simulink model "SWC_FDC_type"  (R2021b)
settings: Solver=FixedStepDiscrete  StartTime=0.0  StopTime=10.0  FixedStep=0.001  RelTol=1e-3
values from neighbouring files (symbols this model uses):
  DID_VCUKey = uint16(0x0202)    [vcu_local_hdr.m]
  DID_XWD = uint16(513)    [vcu_local_hdr.m]
  DIDLen_DKCKey = uint16(8)    [vcu_local_hdr.m]
  DIDLen_DynoMode = uint16(1)    [vcu_local_hdr.m]
  DIDLen_LFLowPresThre = uint16(1)    [vcu_local_hdr.m]
  DIDLen_LFSensorID = uint16(4)    [vcu_local_hdr.m]
  DIDLen_LRLowPresThre = uint16(1)    [vcu_local_hdr.m]
  DIDLen_LRSensorID = uint16(4)    [vcu_local_hdr.m]
  DIDLen_RFLowPresThre = uint16(1)    [vcu_local_hdr.m]
  DIDLen_RFSensorID = uint16(4)    [vcu_local_hdr.m]
  DIDLen_RRLowPresThre = uint16(1)    [vcu_local_hdr.m]
  DIDLen_RRSensorID = uint16(4)    [vcu_local_hdr.m]
  DIDLen_SensorMode = uint16(1)    [vcu_local_hdr.m]
  DIDLen_TPMSLearnSta = uint16(1)    [vcu_local_hdr.m]
  DIDLen_WhlPres = uint16(4)    [vcu_local_hdr.m]
  DIDLen_WhlSensorBattSta = uint16(1)    [vcu_local_hdr.m]
  DIDLen_WhlTmp = uint16(4)    [vcu_local_hdr.m]
  DIDLen_XWDMode = uint16(1)    [vcu_local_hdr.m]
  DIDNum_DKCKey = uint16(0x0202)    [vcu_local_hdr.m]
  DIDNum_DynoMode = uint16(0x0203)    [vcu_local_hdr.m]
  DIDNum_LFLowPresThre = uint16(0x0B08)    [vcu_local_hdr.m]
  DIDNum_LFSensorID = uint16(0x0B01)    [vcu_local_hdr.m]
  DIDNum_LRLowPresThre = uint16(0x0B0A)    [vcu_local_hdr.m]
  DIDNum_LRSensorID = uint16(0x0B03)    [vcu_local_hdr.m]
  DIDNum_RFLowPresThre = uint16(0x0B09)    [vcu_local_hdr.m]
  DIDNum_RFSensorID = uint16(0x0B02)    [vcu_local_hdr.m]
  DIDNum_RRLowPresThre = uint16(0x0B0B)    [vcu_local_hdr.m]
  DIDNum_RRSensorID = uint16(0x0B04)    [vcu_local_hdr.m]
  DIDNum_SensorMode = uint16(0x0B0C)    [vcu_local_hdr.m]
  DIDNum_TPMSLearnSta = uint16(0x0B0D)    [vcu_local_hdr.m]
  DIDNum_WhlPres = uint16(0x0B05)    [vcu_local_hdr.m]
  DIDNum_WhlSensorBattSta = uint16(0x0B07)    [vcu_local_hdr.m]
  DIDNum_WhlTmp = uint16(0x0B06)    [vcu_local_hdr.m]
  DIDNum_XWDMode = uint16(0x0201)    [vcu_local_hdr.m]
  DIDVCUKeyLength = uint16(8)    [vcu_local_hdr.m]
  ENUM_DRIVETRAIN_AWD = uint8(  2  )    [vcu_local_hdr.m]
  ENUM_DRIVETRAIN_FWD = uint8(  1  )    [vcu_local_hdr.m]
  ENUM_DRIVETRAIN_RWD = uint8(  0  )    [vcu_local_hdr.m]
  ENUM_TPMSLearnStatus_LEARNED = uint8(  1  )    [vcu_local_hdr.m]
  ENUM_TPMSLearnStatus_LEARNFAIL = uint8(  2  )    [vcu_local_hdr.m]
  ENUM_TPMSLearnStatus_NOTLEARN = uint8(  0  )    [vcu_local_hdr.m]
  ENUM_TPMSSTA_FAT = uint8(  8  )    [vcu_local_hdr.m]
  ENUM_TPMSSTA_LOWBATTERY = uint8(  2  )    [vcu_local_hdr.m]
  FALSE = boolean( 0 )    [vcu_local_hdr.m]
  ONE_INT = uint8(1)    [vcu_local_hdr.m]
  P_boolean = 0.0    [APPTypes.sldd]
  TRUE = boolean( 1 )    [vcu_local_hdr.m]
  ZERO_FLOAT = single(0)    [vcu_local_hdr.m]
  ZERO_INT = uint8(0)    [vcu_local_hdr.m]
undefined symbols (not defined in the file or in its folder): f32_ApsOutVehSpdSig, KHAL_DKCDecryptEnable_flg_ovrdflg, KHAL_DKCDecryptEnable_flg_ovrdval, KHAL_RandomNumberY1_enum, KHAL_RandomNumberY2_enum, KHAL_RandomNumberY_ovrdflg, KHAL_TPMSRESBUTT_flg_ovrdflg, KHAL_TPMSRESBUTT_flg_ovrdval, R_DIDWriteCDD_CSOP_DIDSet_DKCKey, R_DIDWriteCDD_CSOP_DIDSet_DynoMode, R_DIDWriteCDD_CSOP_DIDSet_LFLowPresThre, R_DIDWriteCDD_CSOP_DIDSet_LFSensorID, R_DIDWriteCDD_CSOP_DIDSet_LRLowPresThre, R_DIDWriteCDD_CSOP_DIDSet_LRSensorID, R_DIDWriteCDD_CSOP_DIDSet_RFLowPresThre, R_DIDWriteCDD_CSOP_DIDSet_RFSensorID, R_DIDWriteCDD_CSOP_DIDSet_RRLowPresThre, R_DIDWriteCDD_CSOP_DIDSet_RRSensorID, R_DIDWriteCDD_CSOP_DIDSet_SensorMode, R_DIDWriteCDD_CSOP_DIDSet_TPMSLearnSta, R_DIDWriteCDD_CSOP_DIDSet_WhlPres, R_DIDWriteCDD_CSOP_DIDSet_WhlSensorBattSta, R_DIDWriteCDD_CSOP_DIDSet_WhlTmp, R_DIDWriteCDD_CSOP_DIDSet_XWDMode, R_E2E_CAN3_VCU1_CSOP_Write_CAN3_VCU1, R_E2E_CAN4_VCU1_CSOP_Write_CAN4_VCU1, R_FDCCDD_Inner_CSOP_FDC_AppCallSleep, R_HALIN_IMU_CSOP_IMUSetSta, R_HALINCDD_CSOP_PAS_Handler, R_HALINCDD_CSOP_UDS_Main, R_HALOUT_APS_CSOP_ApsOutput, R_HALOUTCDD_CSOP_AppNmStateReq, R_HALOUTCDD_CSOP_IVIReset, R_HALOUTCDD_CSOP_SetAcoreRebootCmdACK, R_HALOUTCDD_CSOP_SetSysPwrStat, R_HALOUTCDD_CSOP_SleepRequest, R_NVMReadCDD_Inner_NVM_ReadOperation, R_NVMWriteCDD_Inner_NVM_WriteOperation, R_UDSCDD_CSOP_DdmRestartOperationCycle, R_WDGCDD_CSOP_Call_Watchdog, R_WDGCDD_CSOP_Call_WDG_AppEnd, R_WDGCDD_CSOP_Call_WDG_AppStart, u16_DIDLen_DKCKey, u16_DIDLen_DynoMode, u16_DIDLen_LFLowPresThre, u16_DIDLen_LFSensorID, u16_DIDLen_LRLowPresThre, u16_DIDLen_LRSensorID, u16_DIDLen_RFLowPresThre, u16_DIDLen_RFSensorID, u16_DIDLen_RRLowPresThre, u16_DIDLen_RRSensorID, u16_DIDLen_SensorMode, u16_DIDLen_TPMSLearnSta, u16_DIDLen_WhlPres, u16_DIDLen_WhlSensorBattSta, u16_DIDLen_WhlTmp, u16_DIDLen_XWDMode, u16_DIDNum_DKCKey, u16_DIDNum_DynoMode ... (+42)
libraries: simulink x215, FVT_lib x137, hcu_lib x12, hdlsllib x9, app x1, halin x1, halout x1, inp x1, outp x1
(part 5 of 11)

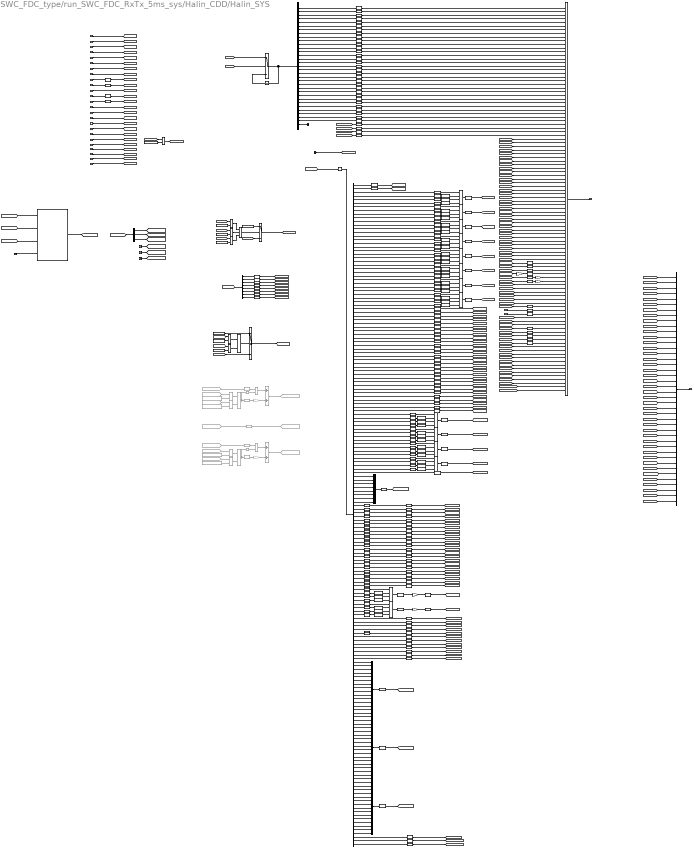
== system SWC_FDC_type/run_SWC_FDC_RxTx_5ms_sys/Halin_CDD/Halin_SYS ==
  note: DID XWD
  note: DID VCUKey
  note: DID APS
  GetSWID_status : Inport
  GetSWID_data : Inport  Port=2
  VHAL_AnyNMID_flg : Inport  Port=3
  VHAL_CurrentNmState_enum : Inport  Port=4
  VHAL_PwrReq_OTA_enum : Inport  Port=5
  VHAL_AllowMovThd_OTA_enum : Inport  Port=6
  VHAL_EvccAplusPwrUpReq_flg : Inport  Port=7
  VHAL_AcoreReadyToSlp_flg : Inport  Port=8
  VHAL_DidXWDSta_flg : Inport  Port=9
  VHAL_DidXWDData_enum : Inport  Port=10
  HAL_NvmReadData_raw : Inport  Port=11
  VHAL_DIDVCUKeyReadSta_flg : Inport  Port=12
  VHAL_GetDIDVCUKey_enum : Inport  Port=13
  VHAL_NvmProtectSta_flg : Inport  Port=14
  VHAL_AuxBattVolmV_100mV : Inport  Port=15
  VHAL_Pedal1Ref5V_raw : Inport  Port=16
  VHAL_Pedal2Ref5V_raw : Inport  Port=17
  VHAL_NetworkReqCalled_flg : Inport  Port=18
  VHAL_PmicBootReason_enum : Inport  Port=19
  VHAL_WisrBootReason_raw32 : Inport  Port=20
  BHAL_DIDGetData_raw : Inport  Port=21
  VHAL_AcoreRebootCmd_raw : Inport  Port=22
  VHAL_CAN1BusOff_raw : Inport  Port=23
  VHAL_CAN2BusOff_raw : Inport  Port=24
  VHAL_CAN3BusOff_raw : Inport  Port=25
  VHAL_CAN4BusOff_raw : Inport  Port=26
  VHAL_CAN5BusOff_raw : Inport  Port=27
  Bitwise OR{1..14} (14 alike) : simulink/Logic and Bit Operations/Bitwise Operator  logicop=OR  UseBitMask=off  NumInputPorts=4  BitMask=bin2dec('00000000000000000000')  BitMaskRealWorld=Stored Integer
  Bus Creator : BusCreator  Inputs=106  OutDataTypeStr=Bus: BHAL_SYS_outputs  NonVirtualBus=on
  Bus Creator4 : BusCreator  Inputs=42
  Bus Selector : BusSelector  OutputSignals=VHAL_DIDGetXWDMode_raw8,VHAL_DIDGetDKCKey_raw8,VHAL_DIDGetDynoMode_raw8
  Constant : Constant  Value=ZERO_INT
  Constant1 : Constant  Value=ONE_INT
  Constant2 : Constant  Value=ZERO_INT
  Constant29 : Constant  Commented=on  Value=ONE_INT
  Constant3 : Constant  Value=ZERO_INT
  Constant30 : Constant  Commented=on  Value=ZERO_INT
  Constant31 : Constant  Commented=on  Value=ONE_INT
  Constant32 : Constant  Commented=on  Value=ZERO_INT
  Constant5 : Constant  Value=ENUM_DRIVETRAIN_FWD
  Constant6 : Constant  Value=ENUM_DRIVETRAIN_RWD
  Constant7 : Constant  Value=ENUM_DRIVETRAIN_AWD
  Constant8 : Constant  Value=ENUM_DRIVETRAIN_RWD
  DIDGet_List : Subsystem
  Data Type Conversion{,3..30,33..44,49..55,98..104,106..107,109,112..121,127,133..135,140,164,187,190..201,208..210,296..297} (92 alike) : DataTypeConversion  OutDataTypeStr=uint8
  Data Type Conversion{1..2,31..32,45..48,56..57,105,108,110..111,122..126,128..132,136..139,141..143,180..185,188..189,211} (40 alike) : DataTypeConversion  OutDataTypeStr=boolean
  Data Type Conversion{58..97,144..163,169..178,186} (71 alike) : DataTypeConversion  OutDataTypeStr=uint32
  Data Type Conversion{165..166,168,179} (4 alike) : DataTypeConversion  OutDataTypeStr=single
  Data Type Conversion167 : DataTypeConversion  OutDataTypeStr=uint16
  Data Type Conversion{203..207} (5 alike) : DataTypeConversion  Commented=on  OutDataTypeStr=uint8
  Demux : Demux  Outputs=33
  Demux1 : Demux  Outputs=182
  Demux2 : Demux  Outputs=8
  Equal{1..5} (5 alike) : RelationalOperator  Operator=~=  OutDataTypeStr=boolean  RndMeth=Simplest
  Equal{20..23} (4 alike) : RelationalOperator  Commented=on  Operator=~=  OutDataTypeStr=boolean  RndMeth=Simplest
  FlashACForceOFF_Verify : Subsystem
  FlashACModeMem_Verify : Subsystem
  FlashAPMDoorControlSta : Subsystem
  FlashAirIntenZone1M_Verify : Subsystem
  FlashCCUSyncSts_Verify : Subsystem
  FlashCountAlarm_Verify : Subsystem
  FlashFaceM_Verify : Subsystem
  FlashFace_Verify : Subsystem
  FlashFootM_Verify : Subsystem
  FlashFoot_Verify : Subsystem
  FlashFrost_Verify : Subsystem
  FlashFuelDoorPos_Verify : Subsystem
  FlashIVIPTGUSStaSW_Verify : Subsystem
  FlashLockSetting_Verify : Subsystem
  FlashMFRDNBrightReq_Verify : Subsystem
  FlashMFSWTri_Verify : Subsystem
  FlashMirrorFlodPos_Verify : Subsystem
  FlashRecAutoFlg_Verify : Subsystem
  FlashRoomLampMode_Verify : Subsystem
  FlashWiperFixMode_Verify : Subsystem
  Flashfdefog_Verify : Subsystem
  FlashsigRecircSt_Verify : Subsystem
  FlashsigSetTempZon1St_Verify : Subsystem
  FlashsigSetTempZon2StM_Verify : Subsystem
  From113 : From  Commented=on  GotoTag=VHAL_DIDGetUSSConfig_raw8
  From114 : From  Commented=on  GotoTag=VHAL_DIDGetTireSize_raw8
  From115 : From  Commented=on  GotoTag=VHAL_DIDGetAPSFunConfig_raw8
  From116 : From  Commented=on  GotoTag=VHAL_DIDGetUSSConfig_raw8
  From117 : From  Commented=on  GotoTag=VHAL_DIDGetUSSConfig_raw8
  From118 : From  Commented=on  GotoTag=VHAL_DIDGetAPSFunConfig_raw8
  From119 : From  Commented=on  GotoTag=VHAL_DIDGetAPSFunConfig_raw8
  Gain : Gain  Gain=5/3788
  Gain1 : Gain  Gain=5/3788
  Gain2 : Gain  Gain=100
  Gain8 : Gain  Commented=on  Gain=0xFF  OutDataTypeStr=uint8
  Gain9 : Gain  Commented=on  Gain=0xFF  OutDataTypeStr=uint8
  Goto140 : Goto  Commented=on  GotoTag=VHAL_USSConfig_raw8
  Goto142 : Goto  Commented=on  GotoTag=VHAL_TireSize_raw8
  Goto143 : Goto  Commented=on  GotoTag=VHAL_APSFunConfig_raw8
  Ground{,2..5} (5 alike) : Ground
  Logical Operator : Logic  Inputs=3  AllPortsSameDT=off  OutDataTypeStr=boolean
  Logical Operator1 : Logic  AllPortsSameDT=off  OutDataTypeStr=boolean
  Multiply1 : Gain  Gain=1/10000
  Multiply2 : Gain  Gain=1/10000
  Mux : Mux  Inputs=8
  Mux1 : Mux  Inputs=16
  Mux2 : Mux  Inputs=16
  Mux3 : Mux  Inputs=16
  NOT : Logic  Commented=on  Operator=NOT  AllPortsSameDT=off  OutDataTypeStr=boolean
  NOT1 : Logic  Commented=on  Operator=NOT  AllPortsSameDT=off  OutDataTypeStr=boolean
  NotEqual : RelationalOperator  Operator=~=  OutDataTypeStr=boolean  RndMeth=Simplest
  OR : Logic  Commented=on  AllPortsSameDT=off  OutDataTypeStr=boolean
  OR1 : Logic  Commented=on  AllPortsSameDT=off  OutDataTypeStr=boolean
  Product : Product  Commented=on
  Product1 : Product  Commented=on
  Selector1 : Selector  InputPortWidth=256  IndexOptions=Index vector (dialog)  Indices=[1:182]  OutputSizes=1
  Shift Arithmetic{1,6,9,12,16,21,25,28..29,32,35..37,40} (14 alike) : ArithShift  BitShiftNumber=8  BitShiftDirection=Left
  Shift Arithmetic{2..3,7,10,13..14,17..18,22,26,30,33,38,41} (14 alike) : ArithShift  BitShiftNumber=16  BitShiftDirection=Left
  Shift Arithmetic{4..5,8,11,15,19..20,23..24,27,31,34,39,42} (14 alike) : ArithShift  BitShiftNumber=24  BitShiftDirection=Left
  Sum : Sum  Commented=on
  Sum1 : Sum  Commented=on
  Switch : Switch  Criteria=u2 ~= 0
  Switch1 : Switch  Criteria=u2 ~= 0
  Switch3 : Switch  Criteria=u2 ~= 0
  Terminator3 : Terminator
  Unit Delay1 : UnitDelay  SampleTime=-1  HasFrameUpgradeWarning=on
  BHAL_SYS_outputs : Outport  OutDataTypeStr=Bus:BHAL_SYS_outputs
  BHAL_SYSTPMS_outputs : Outport  Port=2
  wires:
  Data Type Conversion49/1 -> [VHAL_RFWheelPSW_raw8]  "VHAL_RFWheelPSW_raw8"
  Demux1/36 -> Data Type Conversion46/1
  Data Type Conversion91/1 -> Shift Arithmetic28/1
  Shift Arithmetic29/1 -> Bitwise OR5/2
  Shift Arithmetic14/1 -> Bitwise OR7/3
  Data Type Conversion73/1 -> Bitwise OR7/1
  Data Type Conversion86/1 -> Bitwise OR10/1
  Demux1/39 -> Data Type Conversion51/1
  Demux1/23 -> Data Type Conversion82/1
  Data Type Conversion71/1 -> Shift Arithmetic33/1
  Data Type Conversion48/1 -> [VHAL_RRSensorFail_flg]  "VHAL_RRSensorFail_flg"
  Data Type Conversion90/1 -> Bitwise OR11/1
  Shift Arithmetic18/1 -> Bitwise OR11/3
  [VHAL_EvccAplusPwrUpReq_flg] -> Data Type Conversion32/1
  Demux1/31 -> Data Type Conversion90/1
  Shift Arithmetic26/1 -> Bitwise OR10/3
  Shift Arithmetic32/1 -> Bitwise OR6/2
  Shift Arithmetic15/1 -> Bitwise OR7/4
  Demux1/30 -> Data Type Conversion89/1
  Data Type Conversion53/1 -> [VHAL_RFPindi_enum]  "VHAL_RFPindi_enum"
  Data Type Conversion95/1 -> [VHAL_FlashRFID_raw]  "VHAL_FlashRFID_raw"
  Demux1/7 -> Data Type Conversion65/1
  Ground/1 -> [VHAL_ReadFlashCorrect_flg]  "VHAL_ReadFlashCorrect_flg"
  Data Type Conversion92/1 -> Shift Arithmetic18/1
  Shift Arithmetic17/1 -> Bitwise OR8/3
  Shift Arithmetic16/1 -> Bitwise OR8/2
  Data Type Conversion54/1 -> [VHAL_FlashAntitheft_enum]  "VHAL_FlashAntitheft_enum"
  Shift Arithmetic22/1 -> Bitwise OR9/3
  Demux1/35 -> Data Type Conversion45/1
  Data Type Conversion78/1 -> [VHAL_FlashChkRFID_raw]  "VHAL_FlashChkRFID_raw"
  Shift Arithmetic21/1 -> Bitwise OR9/2
  Demux1/43 -> Data Type Conversion36/1
  Demux1/25 -> Data Type Conversion84/1
  Demux1/44 -> Data Type Conversion53/1
  Bus Creator/1 -> BHAL_SYS_outputs/1
  Demux1/45 -> Data Type Conversion35/1
  Demux1/14 -> Data Type Conversion72/1
  Demux1/29 -> Data Type Conversion88/1
  Demux1/24 -> Data Type Conversion83/1
  Data Type Conversion35/1 -> [VHAL_LRPindi_enum]  "VHAL_LRPindi_enum"
  Demux1/50 -> Data Type Conversion41/1
  GetSWID_status/1 -> [SYSOut]
  Data Type Conversion37/1 -> [VHAL_RRPindi_enum]  "VHAL_RRPindi_enum"
  Demux1/27 -> Data Type Conversion86/1
  Demux1/6 -> Data Type Conversion64/1
  Demux1/3 -> Data Type Conversion59/1
  Data Type Conversion41/1 -> [VHAL_RRP20_raw8]  "VHAL_RRP20_raw8"
  Constant8/1 -> Switch3/1
  Data Type Conversion70/1 -> Shift Arithmetic32/1
  [VHAL_DIDGetXWDMode_raw8] -> Equal1/1
  Data Type Conversion64/1 -> Shift Arithmetic24/1
  Demux1/9 -> Data Type Conversion67/1
  Shift Arithmetic30/1 -> Bitwise OR5/3
  Bitwise OR10/1 -> Data Type Conversion96/1
  Equal2/1 -> Logical Operator/2
  Equal1/1 -> Logical Operator/1
  Switch3/1 -> [VHAL_DrivetrainSelect_enum]  "VHAL_DrivetrainSelect_enum"
  Data Type Conversion45/1 -> [VHAL_LFSensorFail_flg]  "VHAL_LFSensorFail_flg"
  Demux1/32 -> Data Type Conversion91/1
  Switch1/1 -> Unit Delay1/1, Demux/1
  Demux1/46 -> Data Type Conversion37/1
  Shift Arithmetic19/1 -> Bitwise OR11/4
  Demux1/2 -> Data Type Conversion55/1
  Data Type Conversion108/1 -> [VHAL_DIDVCUKeyReadSta_flg]  "VHAL_DIDVCUKeyReadSta_flg"
  Data Type Conversion38/1 -> [VHAL_RFP20_raw8]  "VHAL_RFP20_raw8"
  [VHAL_AcoreReadyToSlp_flg] -> Data Type Conversion1/1
  Demux2/2 -> Data Type Conversion113/1
  Data Type Conversion74/1 -> Shift Arithmetic35/1
  Demux2/5 -> Data Type Conversion116/1
  [VHAL_DIDGetXWDMode_raw8] -> Equal3/1
  Data Type Conversion119/1 -> [VHAL_RandomnumberY_raw8]  "VHAL_RandomnumberY_raw8"
  Demux2/6 -> Data Type Conversion117/1
  Data Type Conversion117/1 -> [VHAL_RandomnumberY_raw6]  "VHAL_RandomnumberY_raw6"
  Data Type Conversion60/1 -> Shift Arithmetic16/1
  Demux1/21 -> Data Type Conversion61/1
  Data Type Conversion114/1 -> [VHAL_RandomnumberY_raw3]  "VHAL_RandomnumberY_raw3"
  Data Type Conversion116/1 -> [VHAL_RandomnumberY_raw5]  "VHAL_RandomnumberY_raw5"
  Demux2/3 -> Data Type Conversion114/1
  Data Type Conversion115/1 -> [VHAL_RandomnumberY_raw4]  "VHAL_RandomnumberY_raw4"
  Shift Arithmetic25/1 -> Bitwise OR10/2
  Data Type Conversion79/1 -> [VHAL_FlashChkLRID_raw]  "VHAL_FlashChkLRID_raw"
  Data Type Conversion81/1 -> Shift Arithmetic20/1
  Data Type Conversion113/1 -> [VHAL_RandomnumberY_raw2]  "VHAL_RandomnumberY_raw2"
  Shift Arithmetic20/1 -> Bitwise OR8/4
  Demux1/11 -> Data Type Conversion69/1
  Data Type Conversion84/1 -> Shift Arithmetic22/1
  Demux1/62 -> Data Type Conversion106/1
  Data Type Conversion94/1 -> [VHAL_FlashLFID_raw]  "VHAL_FlashLFID_raw"
  Demux1/48 -> Data Type Conversion38/1
  Data Type Conversion98/1 -> [VHAL_RFWheelTemp_C]  "VHAL_RFWheelTemp_C"
  Shift Arithmetic12/1 -> Bitwise OR4/2
  Data Type Conversion83/1 -> Shift Arithmetic21/1
  Demux1/49 -> Data Type Conversion39/1
  Demux1/13 -> Data Type Conversion71/1
  Data Type Conversion69/1 -> Bitwise OR6/1
  Demux1/61 -> Data Type Conversion105/1
  Demux1/60 -> Data Type Conversion103/1
  Data Type Conversion104/1 -> [VHAL_Flashchkdatavalid_enum]  "VHAL_Flashchkdatavalid_enum"
  Demux1/59 -> Data Type Conversion104/1
  Bitwise OR7/1 -> Data Type Conversion80/1
  Data Type Conversion103/1 -> [VHAL_Flashdatavalid_enum]  "VHAL_Flashdatavalid_enum"
  Shift Arithmetic23/1 -> Bitwise OR9/4
  Demux1/58 -> Data Type Conversion101/1
  Demux1/20 -> Data Type Conversion60/1
  Data Type Conversion99/1 -> [VHAL_LRWheelTemp_C]  "VHAL_LRWheelTemp_C"
  Demux1/54 -> Data Type Conversion44/1
  Data Type Conversion82/1 -> Bitwise OR9/1
  Demux1/53 -> Data Type Conversion42/1
  Demux1/17 -> Data Type Conversion75/1
  Data Type Conversion96/1 -> [VHAL_FlashLRID_raw]  "VHAL_FlashLRID_raw"
  Demux1/8 -> Data Type Conversion66/1
  Demux1/37 -> Data Type Conversion47/1
  Demux1/34 -> Data Type Conversion93/1
  Demux1/10 -> Data Type Conversion68/1
  Data Type Conversion66/1 -> Shift Arithmetic29/1
  Shift Arithmetic24/1 -> Bitwise OR4/4
  Data Type Conversion50/1 -> [VHAL_LRWheelPSW_raw8]  "VHAL_LRWheelPSW_raw8"
  Data Type Conversion61/1 -> Shift Arithmetic17/1
  Bitwise OR9/1 -> Data Type Conversion95/1
  Data Type Conversion40/1 -> [VHAL_LFP20_raw8]  "VHAL_LFP20_raw8"
  Data Type Conversion112/1 -> [VHAL_RandomnumberY_raw1]  "VHAL_RandomnumberY_raw1"
  Data Type Conversion46/1 -> [VHAL_RFSensorFail_flg]  "VHAL_RFSensorFail_flg"
  Data Type Conversion88/1 -> Shift Arithmetic26/1
  Data Type Conversion67/1 -> Shift Arithmetic30/1
  Data Type Conversion87/1 -> Shift Arithmetic25/1
  Demux1/1 -> Data Type Conversion54/1
  Data Type Conversion127/1 -> [VHAL_FlashAirIntenZone1M_enum]  "VHAL_FlashAirIntenZone1M_enum"
  Demux1/33 -> Data Type Conversion92/1
  Data Type Conversion106/1 -> [VHAL_unlearnSfailvalid_enum]  "VHAL_unlearnSfailvalid_enum"
  Demux1/52 -> Data Type Conversion102/1
  Demux2/1 -> Data Type Conversion112/1
  Data Type Conversion63/1 -> Shift Arithmetic13/1
  Data Type Conversion59/1 -> Bitwise OR4/1
  FlashFaceM_Verify/1(Out1) -> Data Type Conversion125/1
  Data Type Conversion93/1 -> Shift Arithmetic19/1
  Bitwise OR11/1 -> Data Type Conversion97/1
  VHAL_DIDVCUKeyReadSta_flg/1 -> Data Type Conversion108/1
  Bitwise OR5/1 -> Data Type Conversion78/1
  Data Type Conversion43/1 -> [VHAL_LFWheelPress_raw8]  "VHAL_LFWheelPress_raw8"
  Data Type Conversion62/1 -> Shift Arithmetic12/1
  Demux1/40 -> Data Type Conversion49/1
  Demux1/47 -> Data Type Conversion40/1
  Shift Arithmetic28/1 -> Bitwise OR11/2
  Data Type Conversion125/1 -> [VHAL_FlashFaceM_flg]  "VHAL_FlashFaceM_flg"
  Demux1/57 -> Data Type Conversion99/1
  FlashFootM_Verify/1(Out1) -> Data Type Conversion126/1
  Demux1/55 -> Data Type Conversion100/1
  Shift Arithmetic34/1 -> Bitwise OR6/4
  [VHAL_DIDGetDKCKey_raw8] -> Demux2/1
  Demux1/63 -> Data Type Conversion107/1
  Data Type Conversion44/1 -> [VHAL_RRWheelPress_raw8]  "VHAL_RRWheelPress_raw8"
  FlashFoot_Verify/1(Out1) -> Data Type Conversion123/1
  Data Type Conversion100/1 -> [VHAL_LFWheelTemp_C]  "VHAL_LFWheelTemp_C"
  Data Type Conversion36/1 -> [VHAL_LFPindi_enum]  "VHAL_LFPindi_enum"
  Data Type Conversion76/1 -> Shift Arithmetic15/1
  [VHAL_PwrReq_OTA_enum] -> Data Type Conversion29/1
  Data Type Conversion55/1 -> [VHAL_DIDFlashXWDMode_raw8]  "VHAL_FlashDrivetrain_enum"
  Demux1/42 -> Data Type Conversion52/1
  Data Type Conversion121/1 -> [VHAL_FlashACModeMem_enum]  "VHAL_FlashACModeMem_enum"
  Data Type Conversion89/1 -> Shift Arithmetic27/1
  Data Type Conversion72/1 -> Shift Arithmetic34/1
  Data Type Conversion97/1 -> [VHAL_FlashRRID_raw]  "VHAL_FlashRRID_raw"
  Constant6/1 -> Equal2/2
  VHAL_GetDIDVCUKey_enum/1 -> Data Type Conversion109/1
  Data Type Conversion118/1 -> [VHAL_RandomnumberY_raw7]  "VHAL_RandomnumberY_raw7"
  Data Type Conversion85/1 -> Shift Arithmetic23/1
  Demux1/15 -> Data Type Conversion73/1
  [SYSbuffer] -> Switch1/1
  [VHAL_DIDGetXWDMode_raw8] -> Equal2/1
  Data Type Conversion80/1 -> [VHAL_FlashChkRRID_raw]  "VHAL_FlashChkRRID_raw"
  Data Type Conversion123/1 -> [VHAL_FlashFoot_flg]  "VHAL_FlashFoot_flg"
  Demux2/4 -> Data Type Conversion115/1
  Demux1/56 -> Data Type Conversion98/1
  Data Type Conversion132/1 -> [VHAL_Flashfdefog_flg]  "VHAL_Flashfdefog_flg"
  Demux1/5 -> Data Type Conversion63/1
  Data Type Conversion101/1 -> [VHAL_RRWheelTemp_C]  "VHAL_RRWheelTemp_C"
  Data Type Conversion126/1 -> [VHAL_FlashFootM_flg]  "VHAL_FlashFootM_flg"
  Data Type Conversion65/1 -> Bitwise OR5/1
  Demux1/18 -> Data Type Conversion76/1
  Data Type Conversion102/1 -> [VHAL_RFWheelPress_raw8]  "VHAL_RFWheelPress_raw8"
  Data Type Conversion124/1 -> [VHAL_FlashFrost_flg]  "VHAL_FlashFrost_flg"
  [VHAL_DIDGetXWDMode_raw8] -> Switch3/3
  Data Type Conversion68/1 -> Shift Arithmetic31/1
  [SYSOut] -> Switch1/2
  Demux2/7 -> Data Type Conversion118/1
  Unit Delay1/1 -> Switch1/3
  Demux1/16 -> Data Type Conversion74/1
  [VHAL_AllowMovThd_OTA_enum] -> Data Type Conversion30/1
  FlashFrost_Verify/1(Out1) -> Data Type Conversion124/1
  FlashACModeMem_Verify/1(Out1) -> Data Type Conversion121/1
  FlashsigRecircSt_Verify/1(Out1) -> Data Type Conversion130/1
  Demux1/26 -> Data Type Conversion85/1
  Shift Arithmetic35/1 -> Bitwise OR7/2
  Bitwise OR4/1 -> Data Type Conversion77/1
  Flashfdefog_Verify/1(Out1) -> Data Type Conversion132/1
  Logical Operator/1 -> Switch3/2
  Shift Arithmetic33/1 -> Bitwise OR6/3
  FlashACForceOFF_Verify/1(Out1) -> Data Type Conversion129/1
  FlashCCUSyncSts_Verify/1(Out1) -> Data Type Conversion128/1
  FlashAirIntenZone1M_Verify/1(Out1) -> Data Type Conversion127/1
  FlashFace_Verify/1(Out1) -> Data Type Conversion122/1
  Data Type Conversion52/1 -> [VHAL_RRWheelPSW_raw8]  "VHAL_RRWheelPSW_raw8"
  Demux1/51 -> Data Type Conversion43/1
  Shift Arithmetic31/1 -> Bitwise OR5/4
  Data Type Conversion131/1 -> [VHAL_FlashRecAutoFlg_flg]  "VHAL_FlashRecAutoFlg_flg"
  FlashRecAutoFlg_Verify/1(Out1) -> Data Type Conversion131/1
  Bitwise OR8/1 -> Data Type Conversion94/1
  Data Type Conversion129/1 -> [VHAL_FlashACForceOFF_flg]  "VHAL_FlashACForceOFF_flg"
  Selector1/1 -> Demux1/1
  Data Type Conversion39/1 -> [VHAL_LRP20_raw8]  "VHAL_LRP20_raw8"
  Mux/1 -> Data Type Conversion120/1
  Data Type Conversion47/1 -> [VHAL_LRSensorFail_flg]  "VHAL_LRSensorFail_flg"
  Data Type Conversion42/1 -> [VHAL_LRWheelPress_raw8]  "VHAL_LRWheelPress_raw8"
  Demux1/38 -> Data Type Conversion48/1
  Data Type Conversion75/1 -> Shift Arithmetic14/1
  Data Type Conversion105/1 -> [VHAL_unlearnSfali_flg]  "VHAL_unlearnSfali_flg"
  Shift Arithmetic13/1 -> Bitwise OR4/3
  Data Type Conversion107/1 -> [VHAL_Prepresstempvalid_enum]  "VHAL_Prepresstempvalid_enum"
  Data Type Conversion120/1 -> [VHAL_DIDFlashDKCKey_raw8]
  Equal3/1 -> Logical Operator/3
  Bitwise OR6/1 -> Data Type Conversion79/1
  Data Type Conversion58/1 -> Bitwise OR8/1
  Demux1/22 -> Data Type Conversion81/1
  Data Type Conversion130/1 -> [VHAL_FlashsigRecircSt_flg]  "VHAL_FlashsigRecircSt_flg"
  Data Type Conversion51/1 -> [VHAL_LFWheelPSW_raw8]  "VHAL_LFWheelPSW_raw8"
  Data Type Conversion77/1 -> [VHAL_FlashChkLFID_raw]  "VHAL_FlashChkLFID_raw"
  Data Type Conversion109/1 -> [VHAL_GetDIDVCUKey_raw]  "VHAL_GetDIDVCUKey_enum"
  Demux2/8 -> Data Type Conversion119/1
  Data Type Conversion122/1 -> [VHAL_FlashFace_flg]  "VHAL_FlashFace_flg"
  Shift Arithmetic27/1 -> Bitwise OR10/4
  Constant7/1 -> Equal3/2
  Constant5/1 -> Equal1/2
  Data Type Conversion128/1 -> [VHAL_FlashCCUSyncSts_flg]  "VHAL_FlashCCUSyncSts_flg"
  Demux1/4 -> Data Type Conversion62/1
  Demux1/41 -> Data Type Conversion50/1
  Demux1/12 -> Data Type Conversion70/1
  Demux1/28 -> Data Type Conversion87/1
  Demux1/19 -> Data Type Conversion58/1
  GetSWID_data/1 -> [SYSbuffer]
  VHAL_AcoreReadyToSlp_flg/1 -> [VHAL_AcoreReadyToSlp_flg]
  VHAL_AllowMovThd_OTA_enum/1 -> [VHAL_AllowMovThd_OTA_enum]
  VHAL_EvccAplusPwrUpReq_flg/1 -> [VHAL_EvccAplusPwrUpReq_flg]
  VHAL_PwrReq_OTA_enum/1 -> [VHAL_PwrReq_OTA_enum]
  VHAL_AnyNMID_flg/1 -> [VHAL_AnyNMID_flg]
  VHAL_CurrentNmState_enum/1 -> [VHAL_CurrentNmState_enum]
  Data Type Conversion2/1 -> [VHAL_DidXWDSta_flg]  "VHAL_DidXWDSta_flg"
  VHAL_DidXWDSta_flg/1 -> Data Type Conversion2/1
  Data Type Conversion3/1 -> [VHAL_DidXWDData_enum]  "VHAL_DidXWDData_enum"
  VHAL_DidXWDData_enum/1 -> Data Type Conversion3/1
  HAL_NvmReadData_raw/1 -> [HAL_NvmReadData_raw]
  [HAL_NvmReadData_raw] -> Selector1/1
  [VHAL_CurrentNmState_enum] -> Data Type Conversion33/1
  [VHAL_AnyNMID_flg] -> Data Type Conversion31/1
  Data Type Conversion134/1 -> [VHAL_FlashsigSetTempZon2StM_C]  "VHAL_FlashsigSetTempZon2StM_C"
  FlashMFSWTri_Verify/1(Out1) -> Data Type Conversion136/1
  Data Type Conversion142/1 -> [VHAL_FlashWiperFixMode_flg]  "VHAL_FlashWiperFixMode_flg"
  FlashWiperFixMode_Verify/1(Out1) -> Data Type Conversion142/1
  Data Type Conversion143/1 -> [VHAL_FlashIVIPTGUSStaSW_flg]  "VHAL_FlashIVIPTGUSStaSW_flg"
  FlashFuelDoorPos_Verify/1(Out1) -> Data Type Conversion138/1
  FlashIVIPTGUSStaSW_Verify/1(Out1) -> Data Type Conversion143/1
  Data Type Conversion135/1 -> [VHAL_FlashCountAlarm_enum]  "VHAL_FlashCountAlarm_enum"
  Data Type Conversion141/1 -> [VHAL_FlashRoomLampMode_flg]  "VHAL_FlashRoomLampMode_flg"
  FlashRoomLampMode_Verify/1(Out1) -> Data Type Conversion141/1
  FlashMFRDNBrightReq_Verify/1(Out1) -> Data Type Conversion140/1
  Data Type Conversion139/1 -> [VHAL_FlashLockSetting_flg]  "VHAL_FlashLockSetting_flg"
  Data Type Conversion140/1 -> [VHAL_FlashMFRDNBrightReq_pct]  "VHAL_FlashMFRDNBrightReq_pct"
  Data Type Conversion138/1 -> [VHAL_FlashFuelDoorPos_flg]  "VHAL_FlashFuelDoorPos_flg"
  FlashLockSetting_Verify/1(Out1) -> Data Type Conversion139/1
  FlashsigSetTempZon2StM_Verify/1(Out1) -> Data Type Conversion134/1
  Data Type Conversion133/1 -> [VHAL_FlashsigSetTempZon1St_C]  "VHAL_FlashsigSetTempZon1St_C"
  Data Type Conversion136/1 -> [VHAL_FlashMFSWTri_flg]  "VHAL_FlashMFSWTri_flg"
  FlashMirrorFlodPos_Verify/1(Out1) -> Data Type Conversion137/1
  FlashsigSetTempZon1St_Verify/1(Out1) -> Data Type Conversion133/1
  Data Type Conversion137/1 -> [VHAL_FlashMirrorFlodPos_flg]  "VHAL_FlashMirrorFlodPos_flg"
  FlashCountAlarm_Verify/1(Out1) -> Data Type Conversion135/1
  [VHAL_LRP20_raw8] -> Bus Creator4/25
  [VHAL_LRWheelTemp_C] -> Bus Creator4/33
  [VHAL_Flashchkdatavalid_enum] -> Bus Creator4/9
  [VHAL_unlearnSfailvalid_enum] -> Bus Creator4/36
  [VHAL_RRPindi_enum] -> Bus Creator4/22
  [VHAL_FlashS3ID_raw] -> Bus Creator4/40
  [VHAL_LRSensorFail_flg] -> Bus Creator4/13
  [VHAL_FlashLFID_raw] -> Bus Creator4/5
  [VHAL_FlashChkRRID_raw] -> Bus Creator4/4
  [VHAL_FlashIDvaild_enum] -> Bus Creator4/42
  [VHAL_FlashChkRFID_raw] -> Bus Creator4/2
  [VHAL_LFWheelPSW_raw8] -> Bus Creator4/15
  [VHAL_RRWheelPSW_raw8] -> Bus Creator4/18
  [VHAL_RFWheelPress_raw8] -> Bus Creator4/28
  [VHAL_RRWheelPress_raw8] -> Bus Creator4/30
  [VHAL_FlashS2ID_raw] -> Bus Creator4/39
  [VHAL_unlearnSfali_flg] -> Bus Creator4/35
  [VHAL_LFWheelPress_raw8] -> Bus Creator4/27
  [VHAL_RRWheelTemp_C] -> Bus Creator4/34
  [VHAL_LRWheelPress_raw8] -> Bus Creator4/29
  [VHAL_Flashdatavalid_enum] -> Bus Creator4/10
  [VHAL_LFWheelTemp_C] -> Bus Creator4/31
  [VHAL_LFSensorFail_flg] -> Bus Creator4/11
  [VHAL_RRP20_raw8] -> Bus Creator4/26
  [VHAL_Prepresstempvalid_enum] -> Bus Creator4/37
  [VHAL_RFP20_raw8] -> Bus Creator4/24
  [VHAL_FlashRFID_raw] -> Bus Creator4/6
  [VHAL_FlashS4ID_raw] -> Bus Creator4/41
  [VHAL_LRPindi_enum] -> Bus Creator4/21
  Bus Creator4/1 -> BHAL_SYSTPMS_outputs/1
  [VHAL_LRWheelPSW_raw8] -> Bus Creator4/17
  [VHAL_RFPindi_enum] -> Bus Creator4/20
  [VHAL_FlashRRID_raw] -> Bus Creator4/8
  [VHAL_RFSensorFail_flg] -> Bus Creator4/12
  [VHAL_FlashChkLRID_raw] -> Bus Creator4/3
  [VHAL_RRSensorFail_flg] -> Bus Creator4/14
  [VHAL_RFWheelPSW_raw8] -> Bus Creator4/16
  [VHAL_LFP20_raw8] -> Bus Creator4/23
  [VHAL_RFWheelTemp_C] -> Bus Creator4/32
  [VHAL_FlashS1ID_raw] -> Bus Creator4/38
  [VHAL_FlashChkLFID_raw] -> Bus Creator4/1
  [VHAL_FlashLRID_raw] -> Bus Creator4/7
  [VHAL_LFPindi_enum] -> Bus Creator4/19
  Data Type Conversion150/1 -> Shift Arithmetic7/1
  Data Type Conversion156/1 -> Bitwise OR12/1
  Data Type Conversion147/1 -> Shift Arithmetic5/1
  Data Type Conversion151/1 -> Shift Arithmetic8/1
  Data Type Conversion161/1 -> [VHAL_FlashS2ID_raw]  "VHAL_FlashS2ID_raw"
  Demux1/66 -> Data Type Conversion146/1
  Demux1/64 -> Data Type Conversion144/1
  Data Type Conversion158/1 -> Shift Arithmetic3/1
  Demux1/79 -> Data Type Conversion159/1
  Data Type Conversion153/1 -> Shift Arithmetic9/1
  Shift Arithmetic8/1 -> Bitwise OR2/4
  Data Type Conversion144/1 -> Bitwise OR1/1
  Data Type Conversion154/1 -> Shift Arithmetic10/1
  Data Type Conversion159/1 -> Shift Arithmetic4/1
  Shift Arithmetic4/1 -> Bitwise OR12/4
  Demux1/70 -> Data Type Conversion150/1
  Demux1/71 -> Data Type Conversion151/1
  Data Type Conversion148/1 -> Bitwise OR2/1
  Demux1/80 -> Data Type Conversion164/1
  Shift Arithmetic5/1 -> Bitwise OR1/4
  Shift Arithmetic36/1 -> Bitwise OR12/2
  Demux1/68 -> Data Type Conversion148/1
  Shift Arithmetic1/1 -> Bitwise OR1/2
  Demux1/78 -> Data Type Conversion158/1
  Data Type Conversion146/1 -> Shift Arithmetic2/1
  Demux1/67 -> Data Type Conversion147/1
  Shift Arithmetic3/1 -> Bitwise OR12/3
  Data Type Conversion163/1 -> [VHAL_FlashS4ID_raw]  "VHAL_FlashS4ID_raw"
  Demux1/72 -> Data Type Conversion152/1
  Data Type Conversion155/1 -> Shift Arithmetic11/1
  Data Type Conversion160/1 -> [VHAL_FlashS1ID_raw]  "VHAL_FlashS1ID_raw"
  Demux1/69 -> Data Type Conversion149/1
  Bitwise OR12/1 -> Data Type Conversion163/1
  Data Type Conversion157/1 -> Shift Arithmetic36/1
  Bitwise OR1/1 -> Data Type Conversion160/1
  Shift Arithmetic10/1 -> Bitwise OR3/3
  Bitwise OR3/1 -> Data Type Conversion162/1
  Data Type Conversion162/1 -> [VHAL_FlashS3ID_raw]  "VHAL_FlashS3ID_raw"
  Shift Arithmetic7/1 -> Bitwise OR2/3
  Demux1/75 -> Data Type Conversion155/1
  Demux1/74 -> Data Type Conversion154/1
  Shift Arithmetic2/1 -> Bitwise OR1/3
  Data Type Conversion164/1 -> [VHAL_FlashIDvaild_enum]  "VHAL_FlashIDvalid_enum"
  Bitwise OR2/1 -> Data Type Conversion161/1
  Demux1/65 -> Data Type Conversion145/1
  Data Type Conversion149/1 -> Shift Arithmetic6/1
  Data Type Conversion145/1 -> Shift Arithmetic1/1
  Shift Arithmetic6/1 -> Bitwise OR2/2
  Shift Arithmetic11/1 -> Bitwise OR3/4
  Demux1/76 -> Data Type Conversion156/1
  Demux1/73 -> Data Type Conversion153/1
  Data Type Conversion152/1 -> Bitwise OR3/1
  Demux1/77 -> Data Type Conversion157/1
  Shift Arithmetic9/1 -> Bitwise OR3/2
  Demux1/81 -> Mux/1
  Demux1/82 -> Mux/2
  Demux1/83 -> Mux/3
  Demux1/84 -> Mux/4
  Demux1/85 -> Mux/5
  Demux1/86 -> Mux/6
  Demux1/87 -> Mux/7
  Demux1/88 -> Mux/8
  Demux1/89 -> FlashACModeMem_Verify/1(In1)
  Demux1/90 -> FlashFace_Verify/1(In1)
  Demux1/91 -> FlashFoot_Verify/1(In1)
  Demux1/92 -> FlashFrost_Verify/1(In1)
  Demux1/93 -> FlashFaceM_Verify/1(In1)
  Demux1/94 -> FlashFootM_Verify/1(In1)
  Demux1/95 -> FlashCCUSyncSts_Verify/1(In1)
  Demux1/96 -> FlashACForceOFF_Verify/1(In1)
  Demux1/97 -> FlashsigRecircSt_Verify/1(In1)
  Demux1/98 -> FlashRecAutoFlg_Verify/1(In1)
  Demux1/99 -> FlashAirIntenZone1M_Verify/1(In1)
  Demux1/100 -> Flashfdefog_Verify/1(In1)
  Demux1/101 -> FlashsigSetTempZon1St_Verify/1(In1)
  Demux1/102 -> FlashsigSetTempZon2StM_Verify/1(In1)
  Demux1/103 -> FlashCountAlarm_Verify/1(In1)
  Demux1/104 -> FlashMFSWTri_Verify/1(In1)
  Demux1/105 -> FlashMirrorFlodPos_Verify/1(In1)
  Demux1/106 -> FlashFuelDoorPos_Verify/1(In1)
  Demux1/107 -> FlashLockSetting_Verify/1(In1)
  Demux1/108 -> FlashMFRDNBrightReq_Verify/1(In1)
  Demux1/109 -> FlashRoomLampMode_Verify/1(In1)
  Demux1/110 -> FlashWiperFixMode_Verify/1(In1)
  Demux1/111 -> FlashIVIPTGUSStaSW_Verify/1(In1)
  [VHAL_NvmProtectSta_flg] -> Data Type Conversion56/1
  VHAL_NvmProtectSta_flg/1 -> [VHAL_NvmProtectSta_flg]
  Data Type Conversion166/1 -> Gain1/1
  Data Type Conversion165/1 -> Gain/1
  [VHAL_Pedal1Ref5V_raw] -> Data Type Conversion165/1
  [VHAL_Pedal2Ref5V_raw] -> Data Type Conversion166/1
  VHAL_AuxBattVolmV_100mV/1 -> [VHAL_AuxBattVolmV_100mV]
  VHAL_Pedal2Ref5V_raw/1 -> [VHAL_Pedal2Ref5V_raw]
  VHAL_Pedal1Ref5V_raw/1 -> [VHAL_Pedal1Ref5V_raw]
  [VHAL_AuxBattVolmV_100mV] -> Gain2/1
  Demux1/117 -> Data Type Conversion175/1
  Demux1/116 -> Data Type Conversion174/1
  Bitwise OR13/1 -> Data Type Conversion173/1
  Data Type Conversion177/1 -> Shift Arithmetic42/1
  Shift Arithmetic38/1 -> Bitwise OR13/3
  Demux1/114 -> Data Type Conversion171/1
  Shift Arithmetic41/1 -> Bitwise OR14/3
  Demux1/119 -> Data Type Conversion177/1
  Multiply2/1 -> Data Type Conversion168/1
  Data Type Conversion178/1 -> Multiply2/1
  Data Type Conversion175/1 -> Shift Arithmetic40/1
  Data Type Conversion173/1 -> Multiply1/1
  Shift Arithmetic42/1 -> Bitwise OR14/4
  Data Type Conversion176/1 -> Shift Arithmetic41/1
  Demux1/113 -> Data Type Conversion170/1
  Bitwise OR14/1 -> Data Type Conversion178/1
  Shift Arithmetic40/1 -> Bitwise OR14/2
  Data Type Conversion170/1 -> Shift Arithmetic37/1
  Data Type Conversion171/1 -> Shift Arithmetic38/1
  Data Type Conversion174/1 -> Bitwise OR14/1
  Data Type Conversion179/1 -> [VHAL_EAPS1MINMem_pct]  "VHAL_EAPS1MINMem_pct"
  Demux1/118 -> Data Type Conversion176/1
  Shift Arithmetic37/1 -> Bitwise OR13/2
  Demux1/115 -> Data Type Conversion172/1
  Demux1/112 -> Data Type Conversion169/1
  Data Type Conversion169/1 -> Bitwise OR13/1
  Shift Arithmetic39/1 -> Bitwise OR13/4
  Multiply1/1 -> Data Type Conversion179/1
  Data Type Conversion172/1 -> Shift Arithmetic39/1
  Data Type Conversion168/1 -> [VHAL_EAPS2MINMem_pct]  "VHAL_EAPS2MINMem_pct"
  Demux1/120 -> Data Type Conversion180/1
  Demux1/121 -> Data Type Conversion181/1
  Demux1/122 -> Data Type Conversion182/1
  Demux1/123 -> Data Type Conversion183/1
  Data Type Conversion180/1 -> [VHAL_FlashHoodSW_flg]  "VHAL_FlashHoodSW_flg"
  Data Type Conversion181/1 -> [VHAL_FlashTailgateSW_flg]  "VHAL_FlashTailgateSW_flg"
  Data Type Conversion182/1 -> [VHAL_FlashCTDLockSW_flg]  "VHAL_FlashCTDLockSW_flg"
  Data Type Conversion183/1 -> [VHAL_FlashTailgateHDSW_flg]  "VHAL_FlashTailgateHDSW_flg"
  VHAL_NetworkReqCalled_flg/1 -> [VHAL_NetworkReqCalled_flg]
  [VHAL_NetworkReqCalled_flg] -> Data Type Conversion184/1
  Gain2/1 -> Data Type Conversion167/1
  VHAL_PmicBootReason_enum/1 -> Data Type Conversion187/1
  VHAL_WisrBootReason_raw32/1 -> Data Type Conversion186/1
  Demux1/124 -> FlashAPMDoorControlSta/1(In1)
  FlashAPMDoorControlSta/1(Out1) -> Data Type Conversion185/1
  Data Type Conversion185/1 -> [VHAL_FlashAPMDoorControlSta_flg]  "VHAL_FlashAPMDoorControlSta_flg"
  BHAL_DIDGetData_raw/1 -> [BHAL_DIDGetData_raw]
  [BHAL_DIDOrigOutput_raw8] -> Bus Selector/1
  Bus Selector/1 -> [VHAL_DIDGetXWDMode_raw8]  "<VHAL_DIDGetXWDMode_raw8>"
  Bus Selector/2 -> [VHAL_DIDGetDKCKey_raw8]  "<VHAL_DIDGetDKCKey_raw8>"
  VHAL_AcoreRebootCmd_raw/1 -> [VHAL_AcoreRebootCmd_raw]  "VHAL_AcoreRebootCmd_raw"
  Bus Selector/3 -> [VHAL_DIDGetDynoMode_raw8]  "<VHAL_DIDGetDynoMode_raw8>"
  Switch/1 -> [VHAL_DIDGetDynoMode_flg]  "VHAL_DIDGetDynoMode_flg"
  VHAL_CAN1BusOff_raw/1 -> [VHAL_CAN1BusOff_raw]
  VHAL_CAN2BusOff_raw/1 -> [VHAL_CAN2BusOff_raw]
  VHAL_CAN3BusOff_raw/1 -> [VHAL_CAN3BusOff_raw]
  VHAL_CAN4BusOff_raw/1 -> [VHAL_CAN4BusOff_raw]
  VHAL_CAN5BusOff_raw/1 -> [VHAL_CAN5BusOff_raw]
  [VHAL_CAN1BusOff_raw] -> Data Type Conversion57/1
  [VHAL_CAN2BusOff_raw] -> Data Type Conversion110/1
  [VHAL_CAN3BusOff_raw] -> Data Type Conversion188/1
  [VHAL_CAN4BusOff_raw] -> Data Type Conversion111/1
  [VHAL_CAN5BusOff_raw] -> Data Type Conversion189/1
  Constant1/1 -> Equal4/2
  [VHAL_DIDGetDynoMode_raw8] -> Equal4/1
  [VHAL_DIDGetDynoMode_raw8] -> Equal5/1
  Constant2/1 -> Equal5/2
  Equal4/1 -> Logical Operator1/1
  Equal5/1 -> Logical Operator1/2
  Logical Operator1/1 -> Switch/2
  Constant3/1 -> Switch/1
  [VHAL_DIDGetDynoMode_raw8] -> Switch/3
  [VHAL_AcoreRebootCmd_raw] -> NotEqual/1
  Constant/1 -> NotEqual/2
  NotEqual/1 -> [VHAL_AcoreRebootCmd_flg]
  Demux1/131 -> Data Type Conversion190/1
  Demux1/129 -> Data Type Conversion34/1
  Data Type Conversion34/1 -> [VHAL_DIDFlashTurnLampFRThreCurr_raw8]  "VHAL_DIDFlashTurnLampFRThreCurr_raw8"
  Demux1/130 -> Data Type Conversion192/1
  Demux1/128 -> Data Type Conversion191/1
  Demux1/127 -> Data Type Conversion193/1
  Demux1/126 -> Data Type Conversion195/1
  Data Type Conversion192/1 -> [VHAL_DIDFlashTurnLampRLThreCurr_raw8]  "VHAL_DIDFlashTurnLampRLThreCurr_raw8"
  Data Type Conversion195/1 -> [VHAL_DIDFlashDRLDis_raw8]  "VHAL_DIDFlashDRLDis_raw8"
  Data Type Conversion190/1 -> [VHAL_DIDFlashTurnLampRRThreCurr_raw8]  "VHAL_DIDFlashTurnLampRRThreCurr_raw8"
  Data Type Conversion193/1 -> [VHAL_DIDFlashFMHTimer_raw8]  "VHAL_DIDFlashFMHTimer_raw8"
  Demux1/125 -> Data Type Conversion194/1
  Data Type Conversion191/1 -> [VHAL_DIDFlashTurnLampFLThreCurr_raw8]  "VHAL_DIDFlashTurnLampFLThreCurr_raw8"
  Data Type Conversion194/1 -> [VHAL_DIDFlashAutoLock_raw8]  "VHAL_DIDFlashAutoLock_raw8"
  Equal20/1 -> OR/1
  From113/1 -> Equal20/1
  Constant29/1 -> Equal20/2
  From116/1 -> Equal21/1
  Constant30/1 -> Equal21/2
  Equal21/1 -> OR/2
  Data Type Conversion203/1 -> Gain8/1
  OR/1 -> NOT/1, Data Type Conversion203/1
  NOT/1 -> Product/2
  From117/1 -> Data Type Conversion204/1
  Product/1 -> Sum/1
  Gain8/1 -> Sum/2
  Data Type Conversion204/1 -> Product/1
  Sum/1 -> Goto140/1
  Sum1/1 -> Goto143/1
  Data Type Conversion206/1 -> Product1/1
  Gain9/1 -> Sum1/2
  Product1/1 -> Sum1/1
  From115/1 -> Data Type Conversion206/1
  NOT1/1 -> Product1/2
  OR1/1 -> Data Type Conversion205/1, NOT1/1
  Data Type Conversion205/1 -> Gain9/1
  Equal23/1 -> OR1/2
  Constant32/1 -> Equal23/2
  From119/1 -> Equal23/1
  Constant31/1 -> Equal22/2
  From118/1 -> Equal22/1
  Equal22/1 -> OR1/1
  From114/1 -> Data Type Conversion207/1
  Data Type Conversion207/1 -> Goto142/1
  Demux1/132 -> Mux1/1
  Demux1/133 -> Mux1/2
  Demux1/134 -> Mux1/3
  Demux1/135 -> Mux1/4
  Demux1/136 -> Mux1/5
  Demux1/137 -> Mux1/6
  Demux1/138 -> Mux1/7
  Demux1/139 -> Mux1/8
  Demux1/140 -> Mux1/9
  Demux1/141 -> Mux1/10
  Demux1/142 -> Mux1/11
  Demux1/143 -> Mux1/12
  Demux1/144 -> Mux1/13
  Demux1/145 -> Mux1/14
  Demux1/146 -> Mux1/15
  Demux1/147 -> Mux1/16
  Mux1/1 -> Data Type Conversion208/1
  Data Type Conversion208/1 -> [VHAL_DIDFlashUSSConfig_raw8]  "VHAL_DIDFlashUSSConfig_raw8"
  Mux2/1 -> Data Type Conversion209/1
  Demux1/163 -> Mux2/16
  Demux1/162 -> Mux2/15
  Demux1/161 -> Mux2/14
  Demux1/160 -> Mux2/13
  Demux1/159 -> Mux2/12
  Demux1/158 -> Mux2/11
  Demux1/157 -> Mux2/10
  Demux1/156 -> Mux2/9
  Demux1/155 -> Mux2/8
  Demux1/154 -> Mux2/7
  Demux1/153 -> Mux2/6
  Demux1/152 -> Mux2/5
  Demux1/151 -> Mux2/4
  Demux1/150 -> Mux2/3
  Demux1/149 -> Mux2/2
  Demux1/148 -> Mux2/1
  Demux1/164 -> Mux3/1
  Demux1/165 -> Mux3/2
  Demux1/166 -> Mux3/3
  Demux1/167 -> Mux3/4
  Demux1/168 -> Mux3/5
  Demux1/169 -> Mux3/6
  Demux1/170 -> Mux3/7
  Demux1/171 -> Mux3/8
  Demux1/172 -> Mux3/9
  Demux1/173 -> Mux3/10
  Demux1/174 -> Mux3/11
  Demux1/175 -> Mux3/12
  Demux1/176 -> Mux3/13
  Demux1/177 -> Mux3/14
  Demux1/178 -> Mux3/15
  Demux1/179 -> Mux3/16
  Mux3/1 -> Data Type Conversion210/1
  Data Type Conversion209/1 -> [VHAL_DIDFlashTireSize_raw8]  "VHAL_DIDFlashTireSize_raw8"
  Data Type Conversion210/1 -> [VHAL_DIDFlashAPSFunConfig_raw8]  "VHAL_DIDFlashAPSFunConfig_raw8"
  Demux1/180 -> Data Type Conversion211/1
  Data Type Conversion211/1 -> [VHAL_FlashfUnlockSingle_flg]  "VHAL_FlashfUnlockSingle_flg"
  Ground2/1 -> [VHAL_DIDGetUSSConfig_raw8]
  Ground3/1 -> [VHAL_DIDGetTireSize_raw8]
  Ground4/1 -> [VHAL_DIDGetAPSFunConfig_raw8]
  Ground5/1 -> DIDGet_List/4(VHAL_DIDFlashDynoMode_raw8)
  [VHAL_DIDFlashDKCKey_raw8] -> DIDGet_List/3(VHAL_DIDFlashDKCKey_raw8)
  [BHAL_DIDGetData_raw] -> DIDGet_List/1(BHAL_DIDGetData_raw)
  [VHAL_DIDFlashXWDMode_raw8] -> DIDGet_List/2(VHAL_DIDFlashXWDMode_raw8)
  DIDGet_List/1(BHAL_DIDOrigOutput_raw8) -> [BHAL_DIDOrigOutput_raw8]
  Data Type Conversion296/1 -> [VHAL_FlashTPMModelVersion_raw]  "VHAL_FlashTPMModelVersion_raw"
  Data Type Conversion297/1 -> [VHAL_FlashTPMModelVersionChkSum_raw]  "VHAL_FlashTPMModelVersionChkSum_raw"
  Demux1/182 -> Data Type Conversion297/1
  Demux1/181 -> Data Type Conversion296/1
  Demux/18 -> Data Type Conversion198/1
  Demux/1 -> Data Type Conversion/1
  Demux/2 -> Data Type Conversion4/1
  Demux/3 -> Data Type Conversion5/1
  Demux/4 -> Data Type Conversion6/1
  Demux/5 -> Data Type Conversion7/1
  Demux/6 -> Data Type Conversion8/1
  Demux/7 -> Data Type Conversion9/1
  Demux/8 -> Data Type Conversion10/1
  Demux/9 -> Data Type Conversion11/1
  Demux/10 -> Data Type Conversion12/1
  Demux/11 -> Data Type Conversion13/1
  Demux/12 -> Data Type Conversion14/1
  Demux/13 -> Data Type Conversion15/1
  Demux/14 -> Data Type Conversion16/1
  Demux/15 -> Data Type Conversion196/1
  Demux/16 -> Data Type Conversion197/1
  Demux/17 -> Data Type Conversion199/1
  Data Type Conversion/1 -> Bus Creator/1  "VHAL_CarMode1_cnt"
  Data Type Conversion4/1 -> Bus Creator/2  "VHAL_CarModel2_cnt"
  Data Type Conversion5/1 -> Bus Creator/3  "VHAL_CarModel3_cnt"
  Data Type Conversion6/1 -> Bus Creator/4  "VHAL_ECU1_cnt"
  Data Type Conversion7/1 -> Bus Creator/5  "VHAL_ECU2_cnt"
  Data Type Conversion8/1 -> Bus Creator/6  "VHAL_Major1_cnt"
  Data Type Conversion9/1 -> Bus Creator/7  "VHAL_Major2_cnt"
  Data Type Conversion10/1 -> Bus Creator/8  "VHAL_Minor1_cnt"
  Data Type Conversion11/1 -> Bus Creator/9  "VHAL_Minor2_cnt"
  Data Type Conversion12/1 -> Bus Creator/10  "VHAL_Patch1_cnt"
  Data Type Conversion13/1 -> Bus Creator/11  "VHAL_Patch2_cnt"
  Data Type Conversion14/1 -> Bus Creator/12  "VHAL_Country1_cnt"
  Data Type Conversion15/1 -> Bus Creator/13  "VHAL_Country2_cnt"
  Data Type Conversion16/1 -> Bus Creator/14  "VHAL_Variation_cnt"
  Data Type Conversion196/1 -> Bus Creator/15  "VHAL_ECUGen1_cnt"
  Data Type Conversion197/1 -> Bus Creator/16  "VHAL_ECUGen2_cnt"
  Data Type Conversion199/1 -> Bus Creator/17  "VHAL_DrivingMode_cnt"
  Data Type Conversion198/1 -> Bus Creator/18  "VHAL_ModelYear_cnt"
  Data Type Conversion17/1 -> Bus Creator/21  "VHAL_Dash1_cnt"
  Data Type Conversion18/1 -> Bus Creator/22  "VHAL_Change1_cnt"
  Data Type Conversion19/1 -> Bus Creator/23  "VHAL_Change2_cnt"
  Data Type Conversion20/1 -> Bus Creator/24  "VHAL_Dash2_cnt"
  Data Type Conversion21/1 -> Bus Creator/25  "VHAL_SHA1_cnt"
  Data Type Conversion22/1 -> Bus Creator/26  "VHAL_SHA2_cnt"
  Data Type Conversion23/1 -> Bus Creator/27  "VHAL_SHA3_cnt"
  Data Type Conversion24/1 -> Bus Creator/28  "VHAL_SHA4_cnt"
  Data Type Conversion25/1 -> Bus Creator/29  "VHAL_SHA5_cnt"
  Data Type Conversion26/1 -> Bus Creator/30  "VHAL_SHA6_cnt"
  Data Type Conversion27/1 -> Bus Creator/31  "VHAL_SHA7_cnt"
  Data Type Conversion28/1 -> Bus Creator/32  "VHAL_SHA8_cnt"
  Data Type Conversion1/1 -> Bus Creator/33  "VHAL_AcoreReadyToSlp_flg"
  Data Type Conversion29/1 -> Bus Creator/34  "VHAL_PwrReq_OTA_enum"
  Data Type Conversion30/1 -> Bus Creator/35  "VHAL_AllowMovThd_OTA_enum"
  Data Type Conversion32/1 -> Bus Creator/36  "VHAL_EvccAplusPwrUpReq_flg"
  Gain/1 -> Bus Creator/75  "VHAL_Pedal1Ref5V_V"
  Gain1/1 -> Bus Creator/76  "VHAL_Pedal2Ref5V_V"
  Data Type Conversion31/1 -> Bus Creator/71  "VHAL_AnyNMID_flg"
  Data Type Conversion33/1 -> Bus Creator/72  "VHAL_CurrentNmState_enum"
  Data Type Conversion56/1 -> Bus Creator/73  "VHAL_NvmProtectSta_flg"
  Data Type Conversion167/1 -> Bus Creator/74  "VHAL_AuxBattVolmV_mV"
  Data Type Conversion184/1 -> Bus Creator/83  "VHAL_NetworkReqCalled_flg"
  Data Type Conversion187/1 -> Bus Creator/84  "VHAL_PmicBootReason_enum"
  Data Type Conversion186/1 -> Bus Creator/85  "VHAL_WisrBootReason_raw32"
  Data Type Conversion57/1 -> Bus Creator/89  "VHAL_CAN1BusOff_flg"
  Data Type Conversion110/1 -> Bus Creator/90  "VHAL_CAN2BusOff_flg"
  Data Type Conversion188/1 -> Bus Creator/91  "VHAL_CAN3BusOff_flg"
  Data Type Conversion111/1 -> Bus Creator/92  "VHAL_CAN4BusOff_flg"
  Data Type Conversion189/1 -> Bus Creator/93  "VHAL_CAN5BusOff_flg"
  [VHAL_FlashTPMModelVersion_raw] -> Bus Creator/105  "VHAL_FlashTPMModelVersion_raw"
  [VHAL_FlashTPMModelVersionChkSum_raw] -> Bus Creator/106  "VHAL_FlashTPMModelVersionChkSum_raw"
  [VHAL_FlashHoodSW_flg] -> Bus Creator/79
  [VHAL_FlashTailgateSW_flg] -> Bus Creator/80
  [VHAL_FlashCTDLockSW_flg] -> Bus Creator/81
  [VHAL_FlashTailgateHDSW_flg] -> Bus Creator/82
  [VHAL_FlashAPMDoorControlSta_flg] -> Bus Creator/86
  [VHAL_EAPS1MINMem_pct] -> Bus Creator/77
  [VHAL_EAPS2MINMem_pct] -> Bus Creator/78
  [VHAL_DrivetrainSelect_enum] -> Bus Creator/37
  [VHAL_ReadFlashCorrect_flg] -> Bus Creator/38
  [VHAL_FlashAntitheft_enum] -> Bus Creator/39
  [VHAL_RandomnumberY_raw1] -> Bus Creator/40
  [VHAL_RandomnumberY_raw2] -> Bus Creator/41
  [VHAL_RandomnumberY_raw3] -> Bus Creator/42
  [VHAL_RandomnumberY_raw4] -> Bus Creator/43
  [VHAL_RandomnumberY_raw5] -> Bus Creator/44
  [VHAL_RandomnumberY_raw6] -> Bus Creator/45
  [VHAL_RandomnumberY_raw7] -> Bus Creator/46
  [VHAL_RandomnumberY_raw8] -> Bus Creator/47
  [VHAL_FlashACModeMem_enum] -> Bus Creator/48
  [VHAL_FlashFace_flg] -> Bus Creator/49
  [VHAL_FlashFoot_flg] -> Bus Creator/50
  [VHAL_FlashFrost_flg] -> Bus Creator/51
  [VHAL_FlashFaceM_flg] -> Bus Creator/52
  [VHAL_FlashFootM_flg] -> Bus Creator/53
  [VHAL_FlashCCUSyncSts_flg] -> Bus Creator/54
  [VHAL_FlashACForceOFF_flg] -> Bus Creator/55
  [VHAL_FlashsigRecircSt_flg] -> Bus Creator/56
  [VHAL_FlashRecAutoFlg_flg] -> Bus Creator/57
  [VHAL_FlashAirIntenZone1M_enum] -> Bus Creator/58
  [VHAL_Flashfdefog_flg] -> Bus Creator/59
  [VHAL_FlashsigSetTempZon1St_C] -> Bus Creator/60
  [VHAL_FlashsigSetTempZon2StM_C] -> Bus Creator/61
  [VHAL_FlashCountAlarm_enum] -> Bus Creator/62
  [VHAL_FlashMFSWTri_flg] -> Bus Creator/63
  [VHAL_FlashMirrorFlodPos_flg] -> Bus Creator/64
  [VHAL_FlashFuelDoorPos_flg] -> Bus Creator/65
  [VHAL_FlashLockSetting_flg] -> Bus Creator/66
  [VHAL_FlashMFRDNBrightReq_pct] -> Bus Creator/67
  [VHAL_FlashRoomLampMode_flg] -> Bus Creator/68
  [VHAL_FlashWiperFixMode_flg] -> Bus Creator/69
  [VHAL_FlashIVIPTGUSStaSW_flg] -> Bus Creator/70
  [VHAL_AcoreRebootCmd_flg] -> Bus Creator/87  "VHAL_AcoreRebootCmd_flg"
  [VHAL_DIDGetDynoMode_flg] -> Bus Creator/88
  [VHAL_funAuto_flg] -> Bus Creator/94  "VHAL_funAuto_flg"
  [VHAL_DiagDRLOFF_flg] -> Bus Creator/95  "VHAL_DiagDRLOFF_flg"
  [VHAL_DiagFMHT_s] -> Bus Creator/96  "VHAL_DiagFMHT_s"
  [VHAL_DiagFLTC_mA] -> Bus Creator/97  "VHAL_DiagFLTC_mA"
  [VHAL_DiagFRTC_mA] -> Bus Creator/98  "VHAL_DiagFRTC_mA"
  [VHAL_DiagRLTC_mA] -> Bus Creator/99  "VHAL_DiagRLTC_mA"
  [VHAL_DiagRRTC_mA] -> Bus Creator/100  "VHAL_DiagRRTC_mA"
  [VHAL_USSConfig_raw8] -> Bus Creator/101  "VHAL_USSConfig_raw8"
  [VHAL_TireSize_raw8] -> Bus Creator/102  "VHAL_TireSize_raw8"
  [VHAL_APSFunConfig_raw8] -> Bus Creator/103  "VHAL_APSFunConfig_raw8"
  [VHAL_FlashfUnlockSingle_flg] -> Bus Creator/104
  Demux/33 -> Terminator3/1
  Data Type Conversion200/1 -> Bus Creator/19  "VHAL_Var4_cnt"
  Data Type Conversion201/1 -> Bus Creator/20  "VHAL_Var5_cnt"
  Demux/19 -> Data Type Conversion200/1
  Demux/20 -> Data Type Conversion201/1
  Demux/21 -> Data Type Conversion17/1
  Demux/22 -> Data Type Conversion18/1
  Demux/23 -> Data Type Conversion19/1
  Demux/24 -> Data Type Conversion20/1
  Demux/25 -> Data Type Conversion21/1
  Demux/26 -> Data Type Conversion22/1
  Demux/27 -> Data Type Conversion23/1
  Demux/28 -> Data Type Conversion24/1
  Demux/29 -> Data Type Conversion25/1
  Demux/30 -> Data Type Conversion26/1
  Demux/31 -> Data Type Conversion27/1
  Demux/32 -> Data Type Conversion28/1
